simulink model "opv_receiver_HDL_coder_input_Hodgart_Massey"  (R2023a)
settings: Solver=FixedStepDiscrete  StartTime=0.0  StopTime=0.01*(samples_per_frame/sample_rate)  RelTol=1e-3
values from neighbouring files (symbols this model uses):
  bits_per_symbol = 2    [opv.m]
  carrier_frequency = carrier_frequency_multiple_ceil*(orthogonal_frequency)    [opv.m]
  compFilt = design(compSpec,'SystemObject',true)    [opv.m]
  device_clock = 245.76e6    (= 245760000)    [opv.m]
  finalFilt = design(finalSpec,'equiripple','SystemObject',true)    [opv.m]
  intermediateFilt = design(intermediateSpec,'equiripple','SystemObject',true)    [opv.m]
  orthogonal_frequency = 1/(4*bit_period)    (= 13550)    [opv.m]
  symbol_rate = 27100    [opv.m]
undefined symbols (not defined in the file or in its folder): bias, delay, DiscIntNeverNeededParam
libraries: dsphdlfiltering2 x16, hdlsllib x6, dspsrcs4 x4, commrandsrc3 x2, dsphdlsigops2 x2
settings Model: Creator=matt  LastModifiedBy=matt
settings OptimizationCC: BlockReduction=off  ConditionallyExecuteInputs=off  DefaultParameterBehavior=Inlined
settings DebuggingCC: AlgebraicLoopMsg=error
settings HardwareCC: ProdBitPerPointer=32  ProdBitPerSizeT=32  ProdBitPerPtrDiffT=32  ProdLargestAtomicFloat=None  ProdIntDivRoundTo=Undefined  ProdEndianess=Unspecified  ProdWordSize=32  ProdHWDeviceType=ASIC/FPGA->ASIC/FPGA  TargetBitPerLong=64  TargetBitPerPointer=64  TargetBitPerSizeT=64  TargetBitPerPtrDiffT=64  TargetLongLongMode=on  TargetIntDivRoundTo=Zero  TargetEndianess=LittleEndian  TargetWordSize=64  TargetHWDeviceType=Custom Processor->MATLAB Host Computer  ProdEqTarget=off

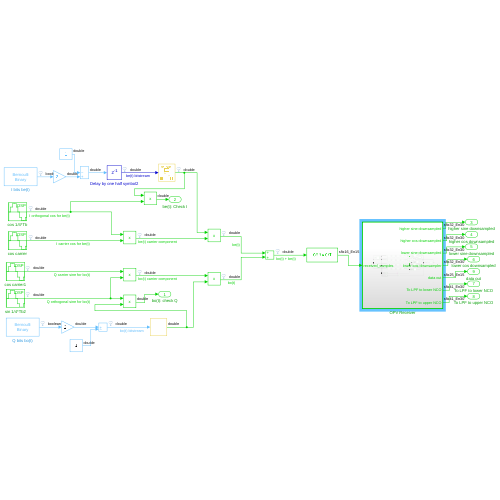
[thumbnail: Simulink's stored preview of the top-level diagram]
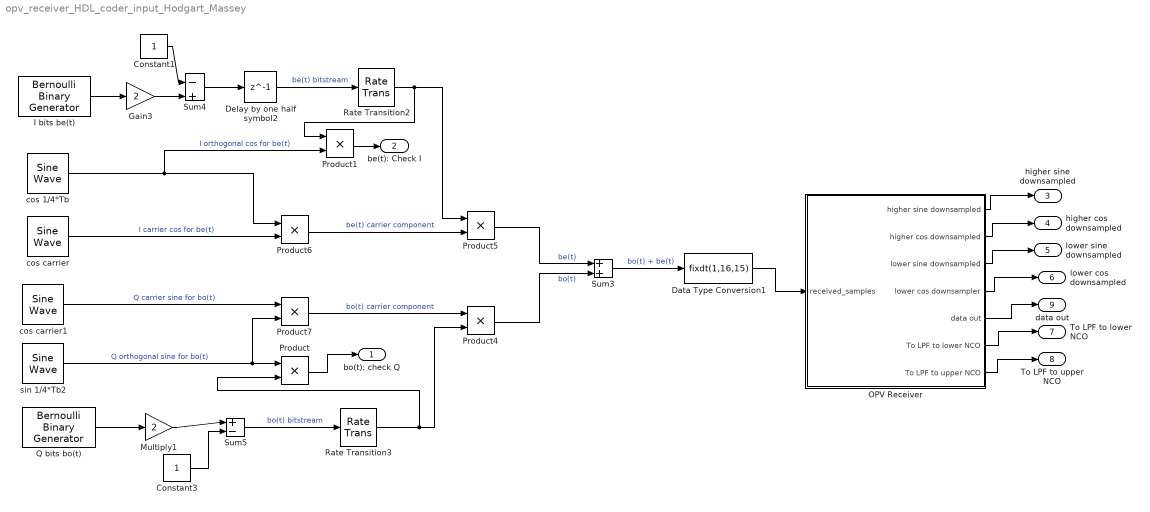
== system opv_receiver_HDL_coder_input_Hodgart_Massey ==
  Constant1 : Constant  OutDataTypeStr=double  SampleTime=1/symbol_rate
  Constant3 : Constant  OutDataTypeStr=double  SampleTime=1/symbol_rate
  Data Type Conversion1 : DataTypeConversion  OutDataTypeStr=fixdt(1,16,15)  SaturateOnIntegerOverflow=off  RndMeth=Floor
  Delay by one half symbol2 : Delay  DelayLength=1  SampleTime=1/(bits_per_symbol*symbol_rate)
  Gain3 : Gain  Gain=2  OutDataTypeStr=double
  I bits be(t) : commrandsrc3/Bernoulli Binary Generator  ProbabilityOfZero=0.5  SeedSource=Auto  Seed=0  SampleTime=1/(symbol_rate)  SamplesPerFrame=1  OutputDataType=boolean  SimulateUsing=Interpreted execution
  Multiply1 : Gain  Gain=2  OutDataTypeStr=double
  OPV Receiver : Subsystem  TreatAsAtomicUnit=on
      settings: LibrarySourceBlock=|
      | hdlsllib/Ports &
      | Subsystems/Subsystem
  Product{,1,4..5} (4 alike) : Product
  Product6 : Product  OutDataTypeStr=double
  Product7 : Product  OutDataTypeStr=double
  Q bits bo(t) : commrandsrc3/Bernoulli Binary Generator  ProbabilityOfZero=0.5  SeedSource=Auto  Seed=0  SampleTime=1/(symbol_rate)  SamplesPerFrame=1  OutputDataType=boolean  SimulateUsing=Interpreted execution
  Rate Transition2 : RateTransition  Deterministic=off  OutPortSampleTimeMultiple=device_clock/symbol_rate  OutPortSampleTime=1/device_clock
  Rate Transition3 : RateTransition  Deterministic=off  OutPortSampleTimeMultiple=device_clock/symbol_rate  OutPortSampleTime=1/device_clock
  Sum3 : Sum  AccumDataTypeStr=double
  Sum4 : Sum  Inputs=|-+  AccumDataTypeStr=double
  Sum5 : Sum  Inputs=|+-  AccumDataTypeStr=double
  cos 1/4*Tb : dspsrcs4/Sine Wave  Amplitude=1  Frequency=orthogonal_frequency  Phase=pi/2  SampleMode=Discrete  OutComplex=Real  CompMethod=Trigonometric fcn  TableSize=Speed  SampleTime=1/device_clock  SamplesPerFrame=1  ResetState=Restart at time zero  OutputFrames=off  dataType=double  wordLen=16  udDataType=sfix(16)  fracBitsMode=User-defined  numFracBits=0  OutDataTypeStr=double  LastOutDataTypeStr=double
  cos carrier : dspsrcs4/Sine Wave  Amplitude=1  Frequency=carrier_frequency  Phase=pi/2  SampleMode=Discrete  OutComplex=Real  CompMethod=Trigonometric fcn  TableSize=Speed  SampleTime=1/device_clock  SamplesPerFrame=1  ResetState=Restart at time zero  OutputFrames=off  dataType=double  wordLen=16  udDataType=sfix(16)  fracBitsMode=User-defined  numFracBits=0  OutDataTypeStr=double  LastOutDataTypeStr=double
  cos carrier1 : dspsrcs4/Sine Wave  Amplitude=1  Frequency=carrier_frequency  Phase=0  SampleMode=Discrete  OutComplex=Real  CompMethod=Trigonometric fcn  TableSize=Speed  SampleTime=1/device_clock  SamplesPerFrame=1  ResetState=Restart at time zero  OutputFrames=off  dataType=double  wordLen=16  udDataType=sfix(16)  fracBitsMode=User-defined  numFracBits=0  OutDataTypeStr=double  LastOutDataTypeStr=double
  sin 1/4*Tb2 : dspsrcs4/Sine Wave  Amplitude=1  Frequency=orthogonal_frequency  Phase=0  SampleMode=Discrete  OutComplex=Real  CompMethod=Trigonometric fcn  TableSize=Speed  SampleTime=1/device_clock  SamplesPerFrame=1  ResetState=Restart at time zero  OutputFrames=off  dataType=double  wordLen=16  udDataType=sfix(16)  fracBitsMode=User-defined  numFracBits=0  OutDataTypeStr=double  LastOutDataTypeStr=double
  bo(t): check Q : Outport
  be(t): Check I : Outport  Port=2
  higher sine downsampled : Outport  Port=3
  higher cos downsampled : Outport  Port=4
  lower sine downsampled : Outport  Port=5
  lower cos downsampled : Outport  Port=6
  To LPF to lower NCO : Outport  Port=7
  To LPF to upper NCO : Outport  Port=8
  data out : Outport  Port=9
  wires:
  sin 1/4*Tb2/1 -> Product7/2, Product/1  "Q orthogonal sine for bo(t)"
  cos carrier1/1 -> Product7/1  "Q carrier sine for bo(t)"
  Sum3/1 -> Data Type Conversion1/1  "bo(t) + be(t)"
  Product6/1 -> Product5/2  "be(t) carrier component"
  Product7/1 -> Product4/1  "bo(t) carrier component"
  cos 1/4*Tb/1 -> Product6/1, Product1/2  "I orthogonal cos for be(t)"
  cos carrier/1 -> Product6/2  "I carrier cos for be(t)"
  Data Type Conversion1/1 -> OPV Receiver/1(received_samples)
  Q bits bo(t)/1 -> Multiply1/1
  Multiply1/1 -> Sum5/1
  Constant3/1 -> Sum5/2
  I bits be(t)/1 -> Gain3/1
  Product4/1 -> Sum3/2  "bo(t)"
  Product5/1 -> Sum3/1  "be(t)"
  Sum4/1 -> Delay by one half symbol2/1
  Rate Transition2/1 -> Product5/1, Product1/1
  Rate Transition3/1 -> Product/2, Product4/2
  Sum5/1 -> Rate Transition3/1  "bo(t) bitstream"
  Gain3/1 -> Sum4/2
  Constant1/1 -> Sum4/1
  Product/1 -> bo(t): check Q/1
  Product1/1 -> be(t): Check I/1
  Delay by one half symbol2/1 -> Rate Transition2/1  "be(t) bitstream"
  OPV Receiver/1(higher sine downsampled) -> higher sine downsampled/1
  OPV Receiver/2(higher cos downsampled) -> higher cos downsampled/1
  OPV Receiver/3(lower sine downsampled) -> lower sine downsampled/1
  OPV Receiver/4(lower cos downsampler) -> lower cos downsampled/1
  OPV Receiver/6(To LPF to lower NCO) -> To LPF to lower NCO/1
  OPV Receiver/7(To LPF to upper NCO) -> To LPF to upper NCO/1
  OPV Receiver/5(data out) -> data out/1

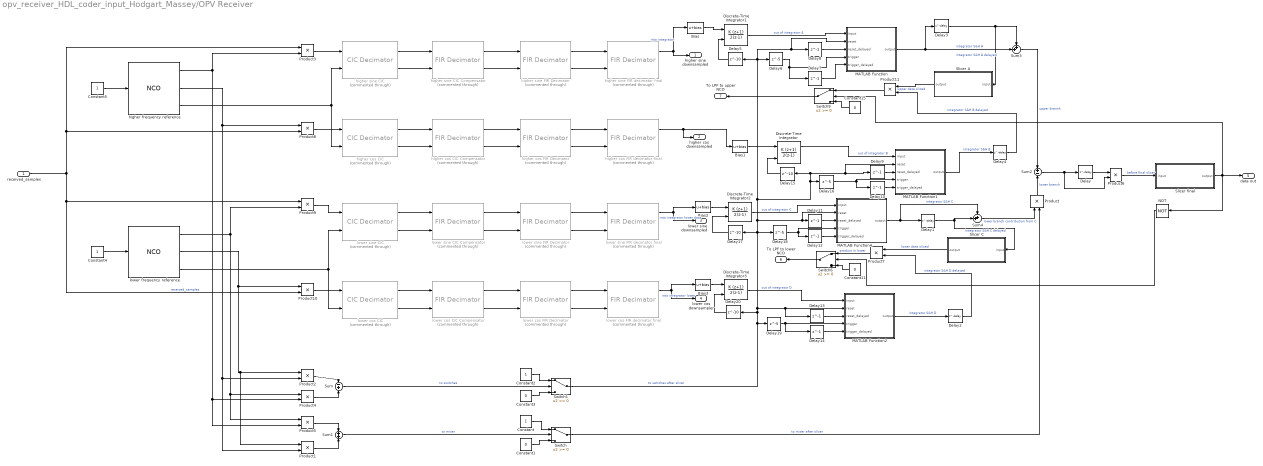
== system opv_receiver_HDL_coder_input_Hodgart_Massey/OPV Receiver ==
  received_samples : Inport
  Bias{,1..3} (4 alike) : Bias  Bias=bias
  Constant : Constant  OutDataTypeStr=fixdt(1,16,15)
  Constant1 : Constant  Value=0  OutDataTypeStr=fixdt(1,16,15)
  Constant11 : Constant  Value=0  OutDataTypeStr=fixdt(1,16,15)
  Constant15 : Constant  Value=0  OutDataTypeStr=fixdt(1,16,15)
  Constant2 : Constant  OutDataTypeStr=boolean
  Constant3 : Constant  Value=0  OutDataTypeStr=boolean
  Constant4 : Constant  OutDataTypeStr=boolean  SampleTime=1/(device_clock)
  Constant5 : Constant  OutDataTypeStr=boolean  SampleTime=1/(device_clock)
  Delay{,1..4} (5 alike) : Delay  DelayLength=delay
  Delay{7..14} (8 alike) : Delay  DelayLength=1
  Delay{5,15,17,20} (4 alike) : Delay  DelayLength=10
  Delay{6,16,18..19} (4 alike) : Delay  DelayLength=5
  Discrete-Time Integrator : DiscreteIntegrator  IntegratorMethod=Accumulation: Trapezoidal  gainval=1/2^9  ExternalReset=rising  SampleTime=-1  OutDataTypeStr=fixdt(1,16,15)  SaturateOnIntegerOverflow=on  LimitOutput=on  UpperSaturationLimit=1  LowerSaturationLimit=-1  ShowSaturationPort=on  ICPrevOutput=DiscIntNeverNeededParam  ICPrevScaledInput=DiscIntNeverNeededParam
  Discrete-Time Integrator1 : DiscreteIntegrator  IntegratorMethod=Accumulation: Trapezoidal  gainval=1/2^9  ExternalReset=rising  SampleTime=-1  OutDataTypeStr=fixdt(1,16,15)  SaturateOnIntegerOverflow=on  LimitOutput=on  UpperSaturationLimit=1  LowerSaturationLimit=-1  ICPrevOutput=DiscIntNeverNeededParam  ICPrevScaledInput=DiscIntNeverNeededParam
  Discrete-Time Integrator2 : DiscreteIntegrator  IntegratorMethod=Accumulation: Trapezoidal  gainval=1/2^9  ExternalReset=rising  SampleTime=-1  OutDataTypeStr=fixdt(1,16,15)  SaturateOnIntegerOverflow=on  LimitOutput=on  UpperSaturationLimit=1  LowerSaturationLimit=-1  ICPrevOutput=DiscIntNeverNeededParam  ICPrevScaledInput=DiscIntNeverNeededParam
  Discrete-Time Integrator3 : DiscreteIntegrator  IntegratorMethod=Accumulation: Trapezoidal  gainval=1/2^9  ExternalReset=rising  SampleTime=-1  OutDataTypeStr=fixdt(1,16,15)  SaturateOnIntegerOverflow=on  LimitOutput=on  UpperSaturationLimit=1  LowerSaturationLimit=-1  ICPrevOutput=DiscIntNeverNeededParam  ICPrevScaledInput=DiscIntNeverNeededParam
  MATLAB Function : MATLAB Function  TreatAsAtomicUnit=on
  MATLAB Function1 : MATLAB Function  TreatAsAtomicUnit=on
  MATLAB Function2 : MATLAB Function  TreatAsAtomicUnit=on
  MATLAB Function4 : MATLAB Function  TreatAsAtomicUnit=on
  NOT : Logic  Operator=NOT  IconShape=distinctive  AllPortsSameDT=off  OutDataTypeStr=fixdt(1,16,15)
  Product{,1..11} (12 alike) : Product
  Slicer A : Subsystem
  Slicer C : Subsystem
  Slicer final : Subsystem
  Sum : Sum  Inputs=-+
  Sum1 : Sum
  Sum2 : Sum  Inputs=+-
  Sum3 : Sum  Inputs=++|
  Sum4 : Sum  Inputs=++|
  Switch{,1,6,9} (4 alike) : Switch  SaturateOnIntegerOverflow=off  InputSameDT=off
  higher cos CIC : dsphdlfiltering2/CIC Decimator  Commented=through  DecimationSource=Property  DecimationFactor=cicParams.DecimationFactor  MaxDecimationFactor=2  DifferentialDelay=cicParams.DifferentialDelay  NumSections=cicParams.NumSections  GainCorrection=on  SimulateUsing=Code generation  OutputDataType=Minimum section word lengths  OutputWordLength=18  ResetInputPort=off  HDLGlobalReset=off
  higher cos CIC Compensator : dsphdlfiltering2/FIR Decimator  Commented=through  Numerator=compFilt.Numerator  FilterStructure=Direct form systolic  DecimationFactor=2  NumCycles=2  SimulateUsing=Code generation  roundingMode=Floor  overflowMode=off  CoefficientsDataTypeStr=Inherit: Same word length as input  OutputDataTypeStr=fixdt(1,18,16)  ResetInputPort=off  HDLGlobalReset=off
  higher cos FIR Decimator : dsphdlfiltering2/FIR Decimator  Commented=through  Numerator=intermediateFilt.Numerator  FilterStructure=Direct form systolic  DecimationFactor=4  NumCycles=8  SimulateUsing=Code generation  roundingMode=Floor  overflowMode=off  CoefficientsDataTypeStr=Inherit: Same word length as input  OutputDataTypeStr=fixdt(1,18,16)  ResetInputPort=off  HDLGlobalReset=off
  higher cos FIR decimator final : dsphdlfiltering2/FIR Decimator  Commented=through  Numerator=finalFilt.Numerator  FilterStructure=Direct form systolic  DecimationFactor=4  NumCycles=16  SimulateUsing=Code generation  roundingMode=Floor  overflowMode=off  CoefficientsDataTypeStr=Inherit: Same word length as input  OutputDataTypeStr=fixdt(1,18,16)  ResetInputPort=off  HDLGlobalReset=off
  higher frequency reference : dsphdlsigops2/NCO  PhaseIncrementSource=Property  PhaseIncrement=phase_increment_higher  PhaseOffsetSource=Property  PhaseOffset=0  DitherSource=None  NumDitherBits=16  SamplesPerFrame=1  LUTCompress=on  ResetAction=off  Waveform=Sine and cosine  PhasePort=off  SimulateUsing=Code generation  AccumulatorWL=32  PhaseQuantization=on  NumQuantizerAccumulatorBits=19  OutputDataType=Binary point scaling  OutputWL=16  OutputFL=15
      settings: LibrarySourceBlock=dsphdlsrcs2/NCO
  higher sine CIC : dsphdlfiltering2/CIC Decimator  Commented=through  DecimationSource=Property  DecimationFactor=cicParams.DecimationFactor  MaxDecimationFactor=2  DifferentialDelay=cicParams.DifferentialDelay  NumSections=cicParams.NumSections  GainCorrection=on  SimulateUsing=Code generation  OutputDataType=Minimum section word lengths  OutputWordLength=18  ResetInputPort=off  HDLGlobalReset=off
  higher sine CIC Compensator : dsphdlfiltering2/FIR Decimator  Commented=through  Numerator=compFilt.Numerator  FilterStructure=Direct form systolic  DecimationFactor=2  NumCycles=2  SimulateUsing=Code generation  roundingMode=Floor  overflowMode=off  CoefficientsDataTypeStr=Inherit: Same word length as input  OutputDataTypeStr=fixdt(1,18,16)  ResetInputPort=off  HDLGlobalReset=off
  higher sine FIR Decimator : dsphdlfiltering2/FIR Decimator  Commented=through  Numerator=intermediateFilt.Numerator  FilterStructure=Direct form systolic  DecimationFactor=4  NumCycles=8  SimulateUsing=Code generation  roundingMode=Floor  overflowMode=off  CoefficientsDataTypeStr=Inherit: Same word length as input  OutputDataTypeStr=fixdt(1,18,16)  ResetInputPort=off  HDLGlobalReset=off
  higher sine FIR decimator final : dsphdlfiltering2/FIR Decimator  Commented=through  Numerator=finalFilt.Numerator  FilterStructure=Direct form systolic  DecimationFactor=4  NumCycles=16  SimulateUsing=Code generation  roundingMode=Floor  overflowMode=off  CoefficientsDataTypeStr=Inherit: Same word length as input  OutputDataTypeStr=fixdt(1,18,16)  ResetInputPort=off  HDLGlobalReset=off
  lower cos CIC : dsphdlfiltering2/CIC Decimator  Commented=through  DecimationSource=Property  DecimationFactor=cicParams.DecimationFactor  MaxDecimationFactor=2  DifferentialDelay=cicParams.DifferentialDelay  NumSections=cicParams.NumSections  GainCorrection=on  SimulateUsing=Code generation  OutputDataType=Minimum section word lengths  OutputWordLength=18  ResetInputPort=off  HDLGlobalReset=off
  lower cos CIC Compensator : dsphdlfiltering2/FIR Decimator  Commented=through  Numerator=compFilt.Numerator  FilterStructure=Direct form systolic  DecimationFactor=2  NumCycles=2  SimulateUsing=Code generation  roundingMode=Floor  overflowMode=off  CoefficientsDataTypeStr=Inherit: Same word length as input  OutputDataTypeStr=fixdt(1,18,16)  ResetInputPort=off  HDLGlobalReset=off
  lower cos FIR Decimator : dsphdlfiltering2/FIR Decimator  Commented=through  Numerator=intermediateFilt.Numerator  FilterStructure=Direct form systolic  DecimationFactor=4  NumCycles=8  SimulateUsing=Code generation  roundingMode=Floor  overflowMode=off  CoefficientsDataTypeStr=Inherit: Same word length as input  OutputDataTypeStr=fixdt(1,18,16)  ResetInputPort=off  HDLGlobalReset=off
  lower cos FIR decimator final : dsphdlfiltering2/FIR Decimator  Commented=through  Numerator=finalFilt.Numerator  FilterStructure=Direct form systolic  DecimationFactor=4  NumCycles=16  SimulateUsing=Code generation  roundingMode=Floor  overflowMode=off  CoefficientsDataTypeStr=Inherit: Same word length as input  OutputDataTypeStr=fixdt(1,18,16)  ResetInputPort=off  HDLGlobalReset=off
  lower frequency reference : dsphdlsigops2/NCO  PhaseIncrementSource=Property  PhaseIncrement=phase_increment_lower  PhaseOffsetSource=Property  PhaseOffset=0  DitherSource=None  NumDitherBits=16  SamplesPerFrame=1  LUTCompress=on  ResetAction=off  Waveform=Sine and cosine  PhasePort=off  SimulateUsing=Code generation  AccumulatorWL=32  PhaseQuantization=on  NumQuantizerAccumulatorBits=19  OutputDataType=Binary point scaling  OutputWL=16  OutputFL=15
      settings: LibrarySourceBlock=dsphdlsrcs2/NCO
  lower sine CIC : dsphdlfiltering2/CIC Decimator  Commented=through  DecimationSource=Property  DecimationFactor=cicParams.DecimationFactor  MaxDecimationFactor=2  DifferentialDelay=cicParams.DifferentialDelay  NumSections=cicParams.NumSections  GainCorrection=on  SimulateUsing=Code generation  OutputDataType=Minimum section word lengths  OutputWordLength=18  ResetInputPort=off  HDLGlobalReset=off
  lower sine CIC Compensator : dsphdlfiltering2/FIR Decimator  Commented=through  Numerator=compFilt.Numerator  FilterStructure=Direct form systolic  DecimationFactor=2  NumCycles=2  SimulateUsing=Code generation  roundingMode=Floor  overflowMode=off  CoefficientsDataTypeStr=Inherit: Same word length as input  OutputDataTypeStr=fixdt(1,18,16)  ResetInputPort=off  HDLGlobalReset=off
  lower sine FIR Decimator : dsphdlfiltering2/FIR Decimator  Commented=through  Numerator=intermediateFilt.Numerator  FilterStructure=Direct form systolic  DecimationFactor=4  NumCycles=8  SimulateUsing=Code generation  roundingMode=Floor  overflowMode=off  CoefficientsDataTypeStr=Inherit: Same word length as input  OutputDataTypeStr=fixdt(1,18,16)  ResetInputPort=off  HDLGlobalReset=off
  lower sine FIR decimator final : dsphdlfiltering2/FIR Decimator  Commented=through  Numerator=finalFilt.Numerator  FilterStructure=Direct form systolic  DecimationFactor=4  NumCycles=16  SimulateUsing=Code generation  roundingMode=Floor  overflowMode=off  CoefficientsDataTypeStr=Inherit: Same word length as input  OutputDataTypeStr=fixdt(1,18,16)  ResetInputPort=off  HDLGlobalReset=off
  higher sine downsampled : Outport
  higher cos downsampled : Outport  Port=2
  lower sine downsampled : Outport  Port=3
  lower cos downsampler : Outport  Port=4
  data out : Outport  Port=5
  To LPF to lower NCO : Outport  Port=6
  To LPF to upper NCO : Outport  Port=7
  wires:
  Constant4/1 -> lower frequency reference/1
  Constant5/1 -> higher frequency reference/1
  higher frequency reference/1 -> Product3/2, Product4/2, Product5/2
  higher frequency reference/2 -> Product8/1, Product1/2, Product2/2
  received_samples/1 -> Product8/2, Product3/1, Product10/2, Product9/1  "received_samples"
  lower frequency reference/1 -> Product5/1, Product4/1, Product9/2
  lower frequency reference/2 -> Product1/1, Product2/1, Product10/1
  higher sine CIC Compensator/2 -> higher sine FIR Decimator/2
  higher sine CIC/1 -> higher sine CIC Compensator/1
  higher sine FIR Decimator/1 -> higher sine FIR decimator final/1
  higher sine FIR Decimator/2 -> higher sine FIR decimator final/2
  higher sine CIC Compensator/1 -> higher sine FIR Decimator/1
  higher sine CIC/2 -> higher sine CIC Compensator/2
  Product3/1 -> higher sine CIC/1
  higher frequency reference/3 -> higher cos CIC/2, higher sine CIC/2
  higher cos CIC Compensator/1 -> higher cos FIR Decimator/1
  higher cos FIR Decimator/1 -> higher cos FIR decimator final/1
  higher cos CIC/1 -> higher cos CIC Compensator/1
  higher cos CIC/2 -> higher cos CIC Compensator/2
  higher cos CIC Compensator/2 -> higher cos FIR Decimator/2
  higher cos FIR Decimator/2 -> higher cos FIR decimator final/2
  Product8/1 -> higher cos CIC/1
  lower cos CIC Compensator/1 -> lower cos FIR Decimator/1
  lower sine FIR Decimator/2 -> lower sine FIR decimator final/2
  lower cos CIC/2 -> lower cos CIC Compensator/2
  lower sine CIC Compensator/2 -> lower sine FIR Decimator/2
  lower cos CIC/1 -> lower cos CIC Compensator/1
  lower sine CIC Compensator/1 -> lower sine FIR Decimator/1
  lower sine CIC/2 -> lower sine CIC Compensator/2
  lower cos FIR Decimator/1 -> lower cos FIR decimator final/1
  lower sine CIC/1 -> lower sine CIC Compensator/1
  lower sine FIR Decimator/1 -> lower sine FIR decimator final/1
  lower cos CIC Compensator/2 -> lower cos FIR Decimator/2
  lower sine FIR decimator final/1 -> Bias2/1, lower sine downsampled/1  "into integrator lower data"
  lower cos FIR Decimator/2 -> lower cos FIR decimator final/2
  Product9/1 -> lower sine CIC/1
  Product10/1 -> lower cos CIC/1
  lower frequency reference/3 -> lower cos CIC/2, lower sine CIC/2
  Product2/1 -> Sum/1
  Product4/1 -> Sum/2
  Product5/1 -> Sum1/1
  Product1/1 -> Sum1/2
  Sum/1 -> Switch1/2  "to switches"
  Sum1/1 -> Switch/2  "to mixer"
  Constant/1 -> Switch/1
  Constant1/1 -> Switch/3
  Constant2/1 -> Switch1/1
  Constant3/1 -> Switch1/3
  Product/1 -> Sum2/2  "lower branch"
  Sum3/1 -> Sum2/1  "upper branch"
  Switch/1 -> Product/2  "to mixer after slicer"
  Sum4/1 -> Product/1  "lower branch contribution from C"
  Sum2/1 -> Product6/2, Delay/1
  Delay/1 -> Product6/1
  Product6/1 -> Slicer final/1(input)  "before final slicer"
  Slicer final/1(output) -> Switch9/2, NOT/1, data out/1
  Delay1/1 -> Sum4/2, Slicer C/1(input)  "integrator S&H C delayed"
  MATLAB Function4/1(output) -> Sum4/1, Delay1/1  "integrator S&H C"
  Switch1/1 -> Delay11/1, MATLAB Function4/2(reset), Delay6/1, Delay5/1, MATLAB Function/2(reset), Delay8/1, Delay9/1, MATLAB Function1/2(reset), Delay15/1, Delay16/1, Delay18/1, Delay17/1, Delay13/1, MATLAB Function2/2(reset), Delay20/1, Delay19/1  "to switches after slicer"
  Delay2/1 -> Product7/2  "integrator S&H D delayed"
  MATLAB Function2/1(output) -> Delay2/1  "integrator S&H D"
  lower cos FIR decimator final/1 -> Bias3/1, lower cos downsampler/1  "into integrator lower"
  Product7/1 -> Switch6/1  "product in lower"
  Constant11/1 -> Switch6/3
  NOT/1 -> Switch6/2
  Switch6/1 -> To LPF to lower NCO/1
  Delay3/1 -> Sum3/1, Slicer A/1(input)  "integrator S&H A delayed"
  Delay4/1 -> Product11/2  "integrator S&H B delayed"
  Product11/1 -> Switch9/1
  Constant15/1 -> Switch9/3
  Slicer A/1(output) -> Product11/1  "upper data sliced"
  Switch9/1 -> To LPF to upper NCO/1
  Discrete-Time Integrator/1 -> MATLAB Function1/1(input)  "out of integrator B"
  MATLAB Function1/1(output) -> Delay4/1  "integrator S&H B"
  higher cos FIR decimator final/1 -> Bias1/1, higher cos downsampled/1
  higher sine FIR decimator final/1 -> Bias/1, higher sine downsampled/1  "into integrator"
  MATLAB Function/1(output) -> Delay3/1, Sum3/2  "integrator S&H A"
  Bias/1 -> Discrete-Time Integrator1/1
  Bias1/1 -> Discrete-Time Integrator/1
  Bias2/1 -> Discrete-Time Integrator2/1
  Discrete-Time Integrator2/1 -> MATLAB Function4/1(input)  "out of integrator C"
  Bias3/1 -> Discrete-Time Integrator3/1
  Discrete-Time Integrator3/1 -> MATLAB Function2/1(input)  "out of integrator D"
  Slicer C/1(output) -> Product7/1  "lower data sliced"
  Discrete-Time Integrator1/1 -> MATLAB Function/1(input)  "out of integrator A"
  Delay7/1 -> MATLAB Function/5(trigger_delayed)
  Delay8/1 -> MATLAB Function/3(reset_delayed)
  Delay5/1 -> Discrete-Time Integrator1/2
  Delay6/1 -> MATLAB Function/4(trigger), Delay7/1
  Delay9/1 -> MATLAB Function1/3(reset_delayed)
  Delay10/1 -> MATLAB Function1/5(trigger_delayed)
  Delay11/1 -> MATLAB Function4/3(reset_delayed)
  Delay12/1 -> MATLAB Function4/5(trigger_delayed)
  Delay13/1 -> MATLAB Function2/3(reset_delayed)
  Delay14/1 -> MATLAB Function2/5(trigger_delayed)
  Delay15/1 -> Discrete-Time Integrator/2
  Delay16/1 -> MATLAB Function1/4(trigger), Delay10/1
  Delay17/1 -> Discrete-Time Integrator2/2
  Delay18/1 -> MATLAB Function4/4(trigger), Delay12/1
  Delay20/1 -> Discrete-Time Integrator3/2
  Delay19/1 -> Delay14/1, MATLAB Function2/4(trigger)

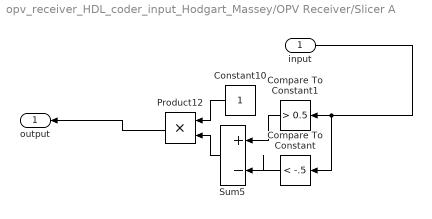
== system opv_receiver_HDL_coder_input_Hodgart_Massey/OPV Receiver/Slicer A ==
  input : Inport
  Compare To Constant : hdlsllib/Logic and Bit Operations/Compare To Constant  relop=<  const=-.5  OutDataTypeStr=uint8
  Compare To Constant1 : hdlsllib/Logic and Bit Operations/Compare To Constant  relop=>  const=0.5  OutDataTypeStr=uint8
  Constant10 : Constant  OutDataTypeStr=fixdt(1,16,15)
  Product12 : Product
  Sum5 : Sum  Inputs=+-|
  output : Outport
  wires:
  input/1 -> Compare To Constant1/1, Compare To Constant/1
  Product12/1 -> output/1
  Compare To Constant1/1 -> Sum5/1
  Sum5/1 -> Product12/2
  Compare To Constant/1 -> Sum5/2
  Constant10/1 -> Product12/1

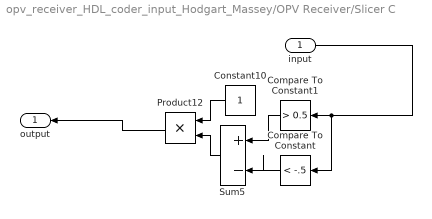
== system opv_receiver_HDL_coder_input_Hodgart_Massey/OPV Receiver/Slicer C ==
  input : Inport
  Compare To Constant : hdlsllib/Logic and Bit Operations/Compare To Constant  relop=<  const=-.5  OutDataTypeStr=uint8
  Compare To Constant1 : hdlsllib/Logic and Bit Operations/Compare To Constant  relop=>  const=0.5  OutDataTypeStr=uint8
  Constant10 : Constant  OutDataTypeStr=fixdt(1,16,15)
  Product12 : Product
  Sum5 : Sum  Inputs=+-|
  output : Outport
  wires:
  Constant10/1 -> Product12/1
  Compare To Constant/1 -> Sum5/2
  Sum5/1 -> Product12/2
  Compare To Constant1/1 -> Sum5/1
  Product12/1 -> output/1
  input/1 -> Compare To Constant/1, Compare To Constant1/1

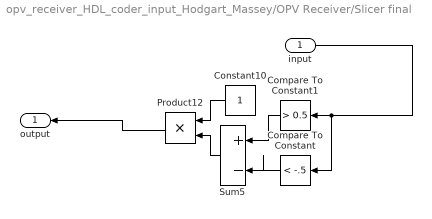
== system opv_receiver_HDL_coder_input_Hodgart_Massey/OPV Receiver/Slicer final ==
  input : Inport
  Compare To Constant : hdlsllib/Logic and Bit Operations/Compare To Constant  relop=<  const=-.5  OutDataTypeStr=uint8
  Compare To Constant1 : hdlsllib/Logic and Bit Operations/Compare To Constant  relop=>  const=0.5  OutDataTypeStr=uint8
  Constant10 : Constant  OutDataTypeStr=fixdt(1,16,15)
  Product12 : Product
  Sum5 : Sum  Inputs=+-|
  output : Outport
  wires:
  Constant10/1 -> Product12/1
  Compare To Constant/1 -> Sum5/2
  Sum5/1 -> Product12/2
  Compare To Constant1/1 -> Sum5/1
  Product12/1 -> output/1
  input/1 -> Compare To Constant/1, Compare To Constant1/1

== matlab function opv_receiver_HDL_coder_input_Hodgart_Massey/OPV Receiver/MATLAB Function1 ==
  data: input input; output output; reset input; reset_delayed input; trigger input; trigger_delayed input
function output   = resettable_sample_and_hold(input, reset, reset_delayed, trigger, trigger_delayed)
%#codegen

%Resettable Sample and Hold Circuit
% This was written because S&H within Resettable Subsystems in Simulink
% is not supported by HDL Coder. We needed this functionality, so this
% custom function was written. 

%possible bug - reset and trigger may need to be reversed. There is
% a glitch. 



initial_value = fi(0,1,16,15);
persistent sample_held;
if isempty(sample_held)
    sample_held = false;
end

persistent output_held_value;
if isempty(output_held_value);
    output_held_value = fi(0,1,16,15);
end


% positive edge detection

positive_reset_edge = and(reset, xor(reset, reset_delayed));
positive_trigger_edge = and(trigger, xor(trigger, trigger_delayed));


switch positive_reset_edge
    case false % not in reset
        switch positive_trigger_edge 
            case false % no trigger yet, continue to hold
                output = output_held_value;
            case true
                if sample_held == false
                    output_held_value = input;
                    output = output_held_value;
                    sample_held = true;
                else
                    output = output_held_value;
                end
            otherwise % we have to cover all the branches
                output = initial_value; 
        end
    case true % reset signal received - arm trigger, continue to hold
        output = output_held_value;
        sample_held = false;
    otherwise % we have to cover all the branches
        output = initial_value;
        
end

== matlab function opv_receiver_HDL_coder_input_Hodgart_Massey/OPV Receiver/MATLAB Function ==
  data: input input; output output; reset input; reset_delayed input; trigger input; trigger_delayed input
function output   = resettable_sample_and_hold(input, reset, reset_delayed, trigger, trigger_delayed)
%#codegen

%Resettable Sample and Hold Circuit
% This was written because S&H within Resettable Subsystems in Simulink
% is not supported by HDL Coder. We needed this functionality, so this
% custom function was written. 

%possible bug - reset and trigger may need to be reversed. There is
% a glitch. 



initial_value = fi(0,1,16,15);
persistent sample_held;
if isempty(sample_held)
    sample_held = false;
end

persistent output_held_value;
if isempty(output_held_value);
    output_held_value = fi(0,1,16,15);
end


% positive edge detection

positive_reset_edge = and(reset, xor(reset, reset_delayed));
positive_trigger_edge = and(trigger, xor(trigger, trigger_delayed));


switch positive_reset_edge
    case false % not in reset
        switch positive_trigger_edge 
            case false % no trigger yet, continue to hold
                output = output_held_value;
            case true
                if sample_held == false
                    output_held_value = input;
                    output = output_held_value;
                    sample_held = true;
                else
                    output = output_held_value;
                end
            otherwise % we have to cover all the branches
                output = initial_value; 
        end
    case true % reset signal received - arm trigger, continue to hold
        output = output_held_value;
        sample_held = false;
    otherwise % we have to cover all the branches
        output = initial_value;
        
end

== matlab function opv_receiver_HDL_coder_input_Hodgart_Massey/OPV Receiver/MATLAB Function2 ==
  data: input input; output output; reset input; reset_delayed input; trigger input; trigger_delayed input
function output   = resettable_sample_and_hold(input, reset, reset_delayed, trigger, trigger_delayed)
%#codegen

%Resettable Sample and Hold Circuit
% This was written because S&H within Resettable Subsystems in Simulink
% is not supported by HDL Coder. We needed this functionality, so this
% custom function was written. 

%possible bug - reset and trigger may need to be reversed. There is
% a glitch. 



initial_value = fi(0,1,16,15);
persistent sample_held;
if isempty(sample_held)
    sample_held = false;
end

persistent output_held_value;
if isempty(output_held_value);
    output_held_value = fi(0,1,16,15);
end


% positive edge detection

positive_reset_edge = and(reset, xor(reset, reset_delayed));
positive_trigger_edge = and(trigger, xor(trigger, trigger_delayed));


switch positive_reset_edge
    case false % not in reset
        switch positive_trigger_edge 
            case false % no trigger yet, continue to hold
                output = output_held_value;
            case true
                if sample_held == false
                    output_held_value = input;
                    output = output_held_value;
                    sample_held = true;
                else
                    output = output_held_value;
                end
            otherwise % we have to cover all the branches
                output = initial_value; 
        end
    case true % reset signal received - arm trigger, continue to hold
        output = output_held_value;
        sample_held = false;
    otherwise % we have to cover all the branches
        output = initial_value;
        
end

== matlab function opv_receiver_HDL_coder_input_Hodgart_Massey/OPV Receiver/MATLAB Function4 ==
  data: input input; output output; reset input; reset_delayed input; trigger input; trigger_delayed input
function output   = resettable_sample_and_hold(input, reset, reset_delayed, trigger, trigger_delayed)
%#codegen

%Resettable Sample and Hold Circuit
% This was written because S&H within Resettable Subsystems in Simulink
% is not supported by HDL Coder. We needed this functionality, so this
% custom function was written. 

%possible bug - reset and trigger may need to be reversed. There is
% a glitch. 



initial_value = fi(0,1,16,15);
persistent sample_held;
if isempty(sample_held)
    sample_held = false;
end

persistent output_held_value;
if isempty(output_held_value);
    output_held_value = fi(0,1,16,15);
end


% positive edge detection

positive_reset_edge = and(reset, xor(reset, reset_delayed));
positive_trigger_edge = and(trigger, xor(trigger, trigger_delayed));


switch positive_reset_edge
    case false % not in reset
        switch positive_trigger_edge 
            case false % no trigger yet, continue to hold
                output = output_held_value;
            case true
                if sample_held == false
                    output_held_value = input;
                    output = output_held_value;
                    sample_held = true;
                else
                    output = output_held_value;
                end
            otherwise % we have to cover all the branches
                output = initial_value; 
        end
    case true % reset signal received - arm trigger, continue to hold
        output = output_held_value;
        sample_held = false;
    otherwise % we have to cover all the branches
        output = initial_value;
        
end
